simulink model "QuadSE3TrajLinFilt"  (R2017b)
settings: Solver=ode4  StartTime=0.0  StopTime=20  FixedStep=sim_step  RelTol=1e-3  EnableMultiTasking=on
values from neighbouring files (symbols this model uses):
  g = 9.81    [initNH.m]
  initlinvel = zeros(3,1)    [initNH.m]
  initpos = zeros(3,1)    [initNH.m]
  initRotMat = eye(3)    [initNH.m]
  initrotvel = zeros(3,1)    [initNH.m]
  J = diag([0.557, 0.557, 1.05]*10e-2)    [initNH.m]
  kd = 1.4*sqrt(4*kp)    [initNH.m]
  kd_z = kd    [initNH.m]
  KDP = 20    [initNH.m]
  KDR = 20    [initNH.m]
  KDY = 10    [initNH.m]
  ki = 1    [initNH.m]
  kp = 15    [initNH.m]
  KPP = 100    [initNH.m]
  KPR = 100    [initNH.m]
  m = 0.5    [initNH.m]
  max_pos_err_norm = 10    [initNH.m]
  max_tilt = 45/180*pi    (= 0.785398163397)    [initNH.m]
settings Model: Creator=Burak  LastModifiedBy=buyue
settings DataIOCC: LimitDataPoints=on  SaveFormat=Array
settings OptimizationCC: LifeSpan=inf
settings DebuggingCC: UnderspecifiedInitializationDetection=Classic  MergeDetectMultiDrivingBlocksExec=none  SolverPrmCheckMsg=warning  StateNameClashWarn=warning  SFUnexpectedBacktrackingDiag=warning  SFNoUnconditionalDefaultTransitionDiag=warning  SFExecutionAtInitializationDiag=none
settings HardwareCC: ProdBitPerPointer=32  ProdBitPerSizeT=32  ProdBitPerPtrDiffT=32  ProdLargestAtomicFloat=None  ProdIntDivRoundTo=Undefined  ProdEndianess=Unspecified  ProdWordSize=32  ProdHWDeviceType=32-bit Generic
settings ModelReferenceCC: PropagateSignalLabelsOutOfModel=off
settings CodeAppCC: StateflowObjectComments=on
settings GRTTargetCC: TargetLangStandard=C89/C90 (ANSI)  GeneratePreprocessorConditionals=Disable all
settings ConfigComp: CovMetricSettings=dw  CovHtmlReporting=on  CovSaveCumulativeToWorkspaceVar=on  CovSaveSingleToWorkspaceVar=on  CovExternalEMLEnable=off

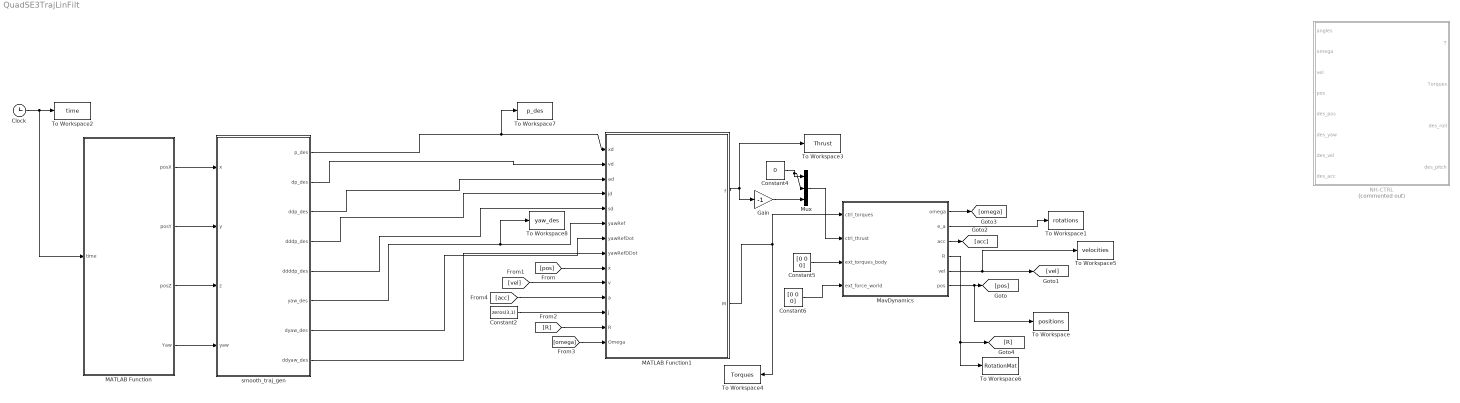
== system QuadSE3TrajLinFilt ==
  Clock : Clock
  Constant2 : Constant  Value=zeros(3,1)
  Constant4 : Constant  Value=0
  Constant5 : Constant  Value=[0 0 0]
  Constant6 : Constant  Value=[0 0 0]
  Gain : Gain  Gain=-1
  MATLAB Function : MATLAB Function  TreatAsAtomicUnit=on
  MATLAB Function1 : MATLAB Function  TreatAsAtomicUnit=on
  MavDynamics : Subsystem
  Mux : Mux  Inputs=3
  NH-CTRL : Subsystem  Commented=on
  To Workspace : ToWorkspace  VariableName=positions  SampleTime=-1
  To Workspace1 : ToWorkspace  VariableName=rotations  SampleTime=-1
  To Workspace2 : ToWorkspace  VariableName=time  SampleTime=-1
  To Workspace3 : ToWorkspace  VariableName=Thrust  SampleTime=-1
  To Workspace4 : ToWorkspace  VariableName=Torques  SampleTime=-1
  To Workspace5 : ToWorkspace  VariableName=velocities  SampleTime=-1
  To Workspace6 : ToWorkspace  VariableName=RotationMat  SampleTime=-1
  To Workspace7 : ToWorkspace  VariableName=p_des  SampleTime=-1
  To Workspace8 : ToWorkspace  VariableName=yaw_des  SampleTime=-1
  smooth_traj_gen : Subsystem
  wires:
  [R] -> MATLAB Function1/13(R)
  [omega] -> MATLAB Function1/14(Omega)
  [pos] -> MATLAB Function1/9(x)
  [vel] -> MATLAB Function1/10(v)
  MATLAB Function1/2(M) -> To Workspace4/1, MavDynamics/1(ctrl_torques)
  MATLAB Function1/1(f) -> Gain/1, To Workspace3/1
  MavDynamics/2(e_a) -> To Workspace1/1
  MavDynamics/5(vel) -> To Workspace5/1, [vel]
  MavDynamics/6(pos) -> To Workspace/1, [pos]
  MavDynamics/1(omega) -> [omega]
  Constant5/1 -> MavDynamics/3(ext_torques_body)
  Constant6/1 -> MavDynamics/4(ext_force_world)
  MavDynamics/4(R) -> [R], To Workspace6/1
  smooth_traj_gen/4(dddp_des) -> MATLAB Function1/4(jd)
  smooth_traj_gen/5(ddddp_des) -> MATLAB Function1/5(sd)
  smooth_traj_gen/7(dyaw_des) -> MATLAB Function1/7(yawRefDot)
  smooth_traj_gen/8(ddyaw_des) -> MATLAB Function1/8(yawRefDDot)
  Clock/1 -> MATLAB Function/1(time), To Workspace2/1
  MATLAB Function/1(posX) -> smooth_traj_gen/1(x)
  MATLAB Function/2(posY) -> smooth_traj_gen/2(y)
  MATLAB Function/3(posZ) -> smooth_traj_gen/3(z)
  MATLAB Function/4(Yaw) -> smooth_traj_gen/4(yaw)
  smooth_traj_gen/3(ddp_des) -> MATLAB Function1/3(ad)
  smooth_traj_gen/2(dp_des) -> MATLAB Function1/2(vd)
  smooth_traj_gen/1(p_des) -> To Workspace7/1, MATLAB Function1/1(xd)
  smooth_traj_gen/6(yaw_des) -> To Workspace8/1, MATLAB Function1/6(yawRef)
  MavDynamics/3(acc) -> [acc]
  [acc] -> MATLAB Function1/11(a)
  Mux/1 -> MavDynamics/2(ctrl_thrust)
  Constant4/1 -> Mux/2, Mux/1
  Gain/1 -> Mux/3
  Constant2/1 -> MATLAB Function1/12(j)

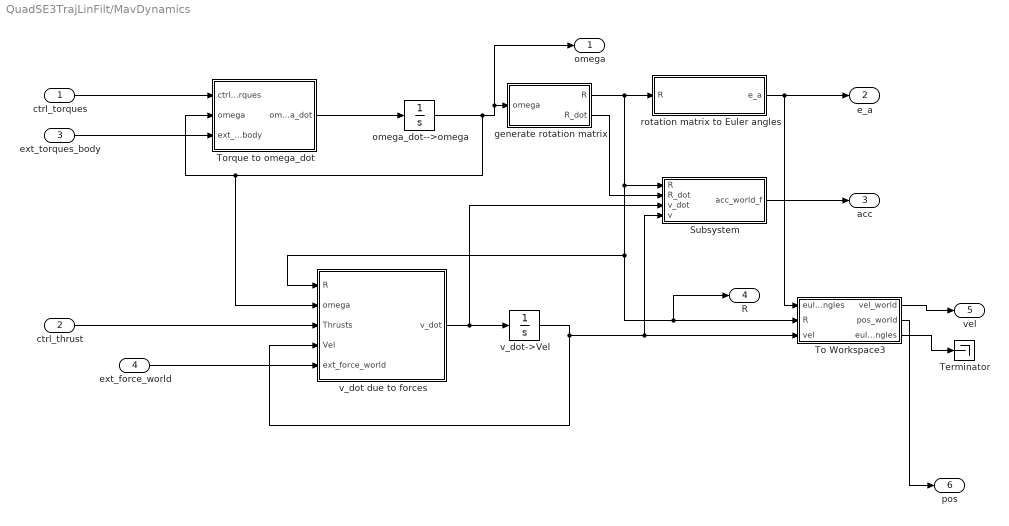
== system QuadSE3TrajLinFilt/MavDynamics ==
  ctrl_torques : Inport
  ctrl_thrust : Inport  Port=2
  ext_torques_body : Inport  Port=3
  ext_force_world : Inport  Port=4
  Subsystem : Subsystem
  Terminator : Terminator
  To Workspace3 : Subsystem
  Torque to omega_dot : Subsystem
  generate rotation matrix : Subsystem
  omega_dot-->omega : Integrator  InitialCondition=initrotvel
  rotation matrix to Euler angles : MATLAB Function  TreatAsAtomicUnit=on
  v_dot due to forces : Subsystem
  v_dot->Vel : Integrator  InitialCondition=initlinvel
  omega : Outport
  e_a : Outport  Port=2
  acc : Outport  Port=3
  R : Outport  Port=4
  vel : Outport  Port=5
  pos : Outport  Port=6
  wires:
  To Workspace3/3("euler_angles ") -> Terminator/1
  v_dot due to forces/1(v_dot) -> Subsystem/3(v_dot), v_dot->Vel/1
  omega_dot-->omega/1 -> v_dot due to forces/2(omega), Torque to omega_dot/2(omega), omega/1, generate rotation matrix/1(omega)
  ext_force_world/1 -> v_dot due to forces/5(ext_force_world)
  To Workspace3/2(pos_world) -> pos/1
  Subsystem/1(acc_world_f) -> acc/1
  To Workspace3/1(vel_world) -> vel/1
  ctrl_thrust/1 -> v_dot due to forces/3(Thrusts)
  rotation matrix to Euler angles/1(e_a) -> e_a/1, To Workspace3/1(euler_angles)
  ext_torques_body/1 -> Torque to omega_dot/3(ext_torques_body)
  Torque to omega_dot/1(omega_dot) -> omega_dot-->omega/1
  generate rotation matrix/1(R) -> rotation matrix to Euler angles/1(R), R/1, To Workspace3/2(R), v_dot due to forces/1(R), Subsystem/1(R)
  v_dot->Vel/1 -> To Workspace3/3(vel), Subsystem/4(v), v_dot due to forces/4(Vel)
  generate rotation matrix/2(R_dot) -> Subsystem/2(R_dot)
  ctrl_torques/1 -> Torque to omega_dot/1(ctrl_orques)

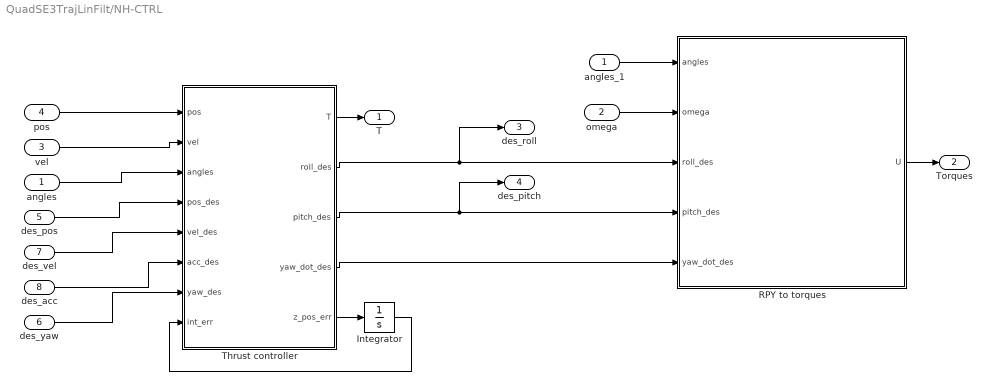
== system QuadSE3TrajLinFilt/NH-CTRL ==
  angles : Inport
  omega : Inport  Port=2
  vel : Inport  Port=3
  pos : Inport  Port=4
  des_pos : Inport  Port=5
  des_yaw : Inport  Port=6
  des_vel : Inport  Port=7
  des_acc : Inport  Port=8
  Integrator : Integrator
  RPY to torques : MATLAB Function  TreatAsAtomicUnit=on
  Thrust controller : MATLAB Function  TreatAsAtomicUnit=on
  angles_1 : InportShadow
  T : Outport
  Torques : Outport  Port=2
  des_roll : Outport  Port=3
  des_pitch : Outport  Port=4
  wires:
  Integrator/1 -> Thrust controller/8(int_err)
  omega/1 -> RPY to torques/2(omega)
  vel/1 -> Thrust controller/2(vel)
  Thrust controller/3(pitch_des) -> des_pitch/1, RPY to torques/4(pitch_des)
  Thrust controller/4(yaw_dot_des) -> RPY to torques/5(yaw_dot_des)
  angles_1/1 -> RPY to torques/1(angles)
  des_acc/1 -> Thrust controller/6(acc_des)
  des_pos/1 -> Thrust controller/4(pos_des)
  des_yaw/1 -> Thrust controller/7(yaw_des)
  pos/1 -> Thrust controller/1(pos)
  Thrust controller/2(roll_des) -> des_roll/1, RPY to torques/3(roll_des)
  angles/1 -> Thrust controller/3(angles)
  Thrust controller/5(z_pos_err) -> Integrator/1
  des_vel/1 -> Thrust controller/5(vel_des)
  RPY to torques/1(U) -> Torques/1
  Thrust controller/1(T) -> T/1

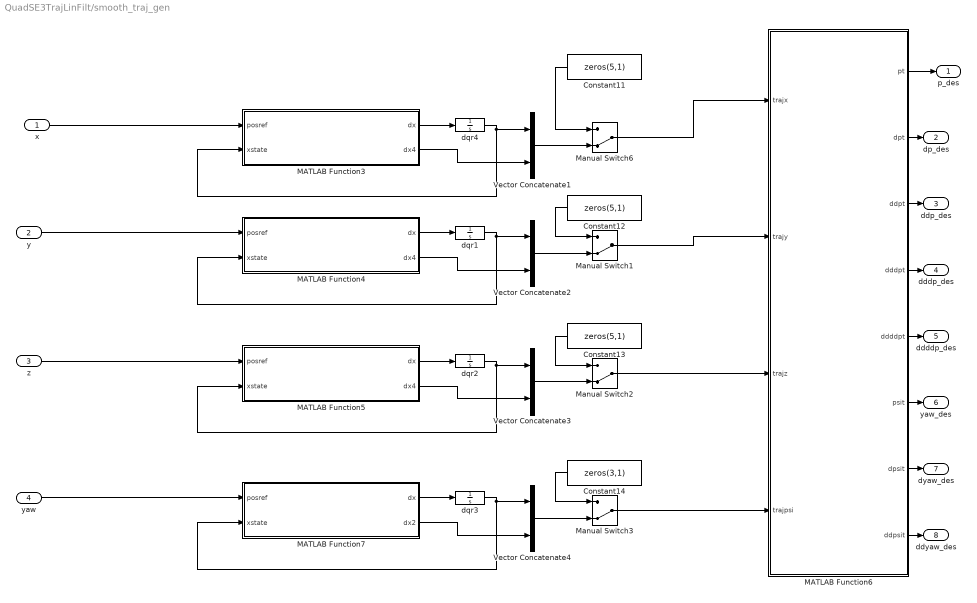
== system QuadSE3TrajLinFilt/smooth_traj_gen ==
  x : Inport
  y : Inport  Port=2
  z : Inport  Port=3
  yaw : Inport  Port=4
  Constant11 : Constant  Value=zeros(5,1)
  Constant12 : Constant  Value=zeros(5,1)
  Constant13 : Constant  Value=zeros(5,1)
  Constant14 : Constant  Value=zeros(3,1)
  MATLAB Function3 : MATLAB Function  TreatAsAtomicUnit=on
  MATLAB Function4 : MATLAB Function  TreatAsAtomicUnit=on
  MATLAB Function5 : MATLAB Function  TreatAsAtomicUnit=on
  MATLAB Function6 : MATLAB Function  TreatAsAtomicUnit=on
  MATLAB Function7 : MATLAB Function  TreatAsAtomicUnit=on
  Manual Switch{1..3,6} (4 alike) : ManualSwitch  CurrentSetting=0
  Vector Concatenate{1..4} (4 alike) : Concatenate
  dqr1 : Integrator  InitialCondition=[0,0,0,0];
  dqr2 : Integrator  InitialCondition=[0,0,0,0];
  dqr3 : Integrator  InitialCondition=[0,0];
  dqr4 : Integrator  InitialCondition=[0,0,0,0];
  p_des : Outport
  dp_des : Outport  Port=2
  ddp_des : Outport  Port=3
  dddp_des : Outport  Port=4
  ddddp_des : Outport  Port=5
  yaw_des : Outport  Port=6
  dyaw_des : Outport  Port=7
  ddyaw_des : Outport  Port=8
  wires:
  MATLAB Function6/1(pt) -> p_des/1
  MATLAB Function7/2(dx2) -> Vector Concatenate4/2
  x/1 -> MATLAB Function3/1(posref)
  dqr2/1 -> Vector Concatenate3/1, MATLAB Function5/2(xstate)
  MATLAB Function3/1(dx) -> dqr4/1
  MATLAB Function7/1(dx) -> dqr3/1
  yaw/1 -> MATLAB Function7/1(posref)
  MATLAB Function5/2(dx4) -> Vector Concatenate3/2
  Constant14/1 -> Manual Switch3/1
  Manual Switch3/1 -> MATLAB Function6/4(trajpsi)
  MATLAB Function4/1(dx) -> dqr1/1
  MATLAB Function3/2(dx4) -> Vector Concatenate1/2
  MATLAB Function5/1(dx) -> dqr2/1
  Constant13/1 -> Manual Switch2/1
  MATLAB Function4/2(dx4) -> Vector Concatenate2/2
  Vector Concatenate2/1 -> Manual Switch1/2
  Vector Concatenate1/1 -> Manual Switch6/2
  Constant11/1 -> Manual Switch6/1
  Vector Concatenate3/1 -> Manual Switch2/2
  Manual Switch6/1 -> MATLAB Function6/1(trajx)
  Constant12/1 -> Manual Switch1/1
  Manual Switch1/1 -> MATLAB Function6/2(trajy)
  y/1 -> MATLAB Function4/1(posref)
  z/1 -> MATLAB Function5/1(posref)
  dqr3/1 -> Vector Concatenate4/1, MATLAB Function7/2(xstate)
  dqr4/1 -> Vector Concatenate1/1, MATLAB Function3/2(xstate)
  dqr1/1 -> Vector Concatenate2/1, MATLAB Function4/2(xstate)
  Vector Concatenate4/1 -> Manual Switch3/2
  Manual Switch2/1 -> MATLAB Function6/3(trajz)
  MATLAB Function6/4(dddpt) -> dddp_des/1
  MATLAB Function6/2(dpt) -> dp_des/1
  MATLAB Function6/5(ddddpt) -> ddddp_des/1
  MATLAB Function6/6(psit) -> yaw_des/1
  MATLAB Function6/8(ddpsit) -> ddyaw_des/1
  MATLAB Function6/7(dpsit) -> dyaw_des/1
  MATLAB Function6/3(ddpt) -> ddp_des/1

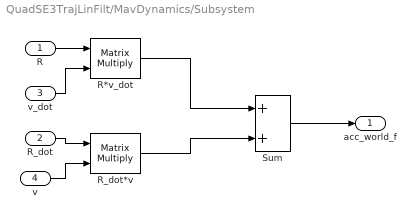
== system QuadSE3TrajLinFilt/MavDynamics/Subsystem ==
  R : Inport
  R_dot : Inport  Port=2
  v_dot : Inport  Port=3
  v : Inport  Port=4
  R*v_dot : Product  Multiplication=Matrix(*)  RndMeth=Zero
  R_dot*v : Product  Multiplication=Matrix(*)  RndMeth=Zero
  Sum : Sum
  acc_world_f : Outport
  wires:
  Sum/1 -> acc_world_f/1
  R/1 -> R*v_dot/1
  v_dot/1 -> R*v_dot/2
  R_dot/1 -> R_dot*v/1
  v/1 -> R_dot*v/2
  R*v_dot/1 -> Sum/1
  R_dot*v/1 -> Sum/2

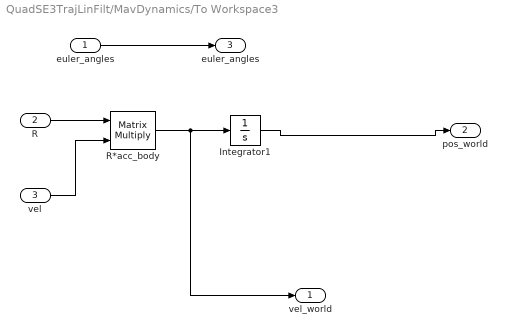
== system QuadSE3TrajLinFilt/MavDynamics/To Workspace3 ==
  euler_angles : Inport
  R : Inport  Port=2
  vel : Inport  Port=3
  Integrator1 : Integrator  InitialCondition=initpos
  R*acc_body : Product  Multiplication=Matrix(*)  RndMeth=Zero
  vel_world : Outport
  pos_world : Outport  Port=2
  "euler_angles " : Outport  Port=3
  wires:
  R/1 -> R*acc_body/1
  vel/1 -> R*acc_body/2
  euler_angles/1 -> "euler_angles "/1
  R*acc_body/1 -> vel_world/1, Integrator1/1
  Integrator1/1 -> pos_world/1

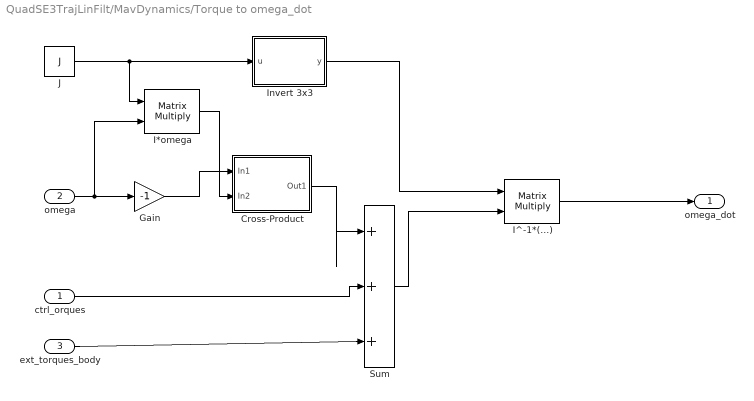
== system QuadSE3TrajLinFilt/MavDynamics/Torque to omega_dot ==
  ctrl_orques : Inport
  omega : Inport  Port=2
  ext_torques_body : Inport  Port=3
  Cross-Product : Subsystem
  Gain : Gain  Gain=-1
  I*omega : Product  Multiplication=Matrix(*)  RndMeth=Zero
  I^-1*(...) : Product  Multiplication=Matrix(*)  RndMeth=Zero
  Invert 3x3 : MATLAB Function  TreatAsAtomicUnit=on
  J : Constant  Value=J
  Sum : Sum  Inputs=|+++
  omega_dot : Outport
  wires:
  omega/1 -> I*omega/2, Gain/1
  J/1 -> I*omega/1, Invert 3x3/1(u)
  I*omega/1 -> Cross-Product/2(In2)
  Invert 3x3/1(y) -> I^-1*(...)/1
  I^-1*(...)/1 -> omega_dot/1
  ctrl_orques/1 -> Sum/2
  Sum/1 -> I^-1*(...)/2
  Gain/1 -> Cross-Product/1(In1)
  Cross-Product/1(Out1) -> Sum/1
  ext_torques_body/1 -> Sum/3

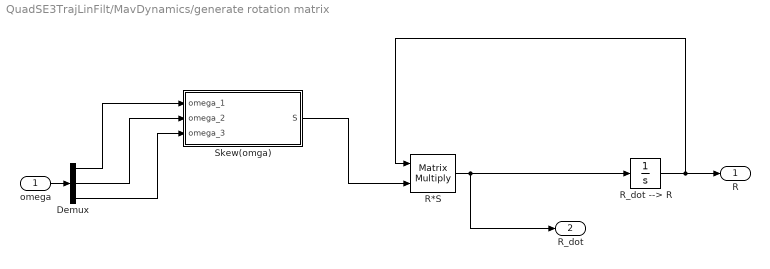
== system QuadSE3TrajLinFilt/MavDynamics/generate rotation matrix ==
  omega : Inport
  Demux : Demux  Outputs=3
  R*S : Product  Multiplication=Matrix(*)  RndMeth=Zero
  R_dot --> R : Integrator  InitialCondition=initRotMat
  Skew(omga) : MATLAB Function  TreatAsAtomicUnit=on
  R : Outport
  R_dot : Outport  Port=2
  wires:
  R*S/1 -> R_dot --> R/1, R_dot/1
  R_dot --> R/1 -> R/1, R*S/1
  omega/1 -> Demux/1
  Demux/1 -> Skew(omga)/1(omega_1)
  Demux/2 -> Skew(omga)/2(omega_2)
  Demux/3 -> Skew(omga)/3(omega_3)
  Skew(omga)/1(S) -> R*S/2

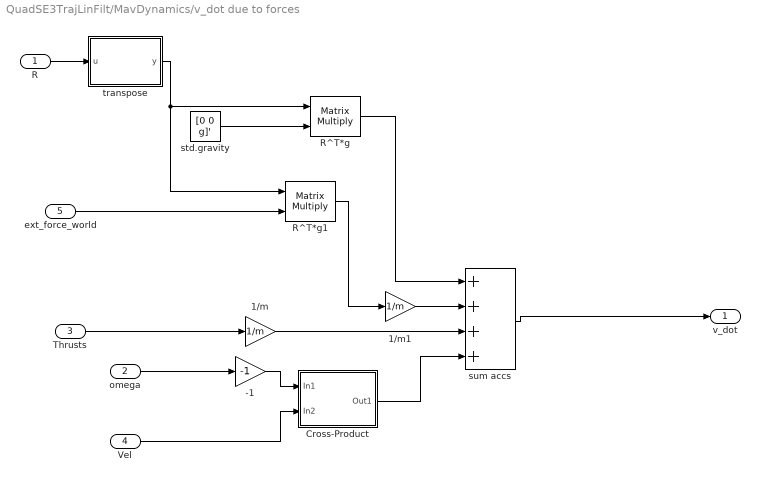
== system QuadSE3TrajLinFilt/MavDynamics/v_dot due to forces ==
  R : Inport
  omega : Inport  Port=2
  Thrusts : Inport  Port=3
  Vel : Inport  Port=4
  ext_force_world : Inport  Port=5
  -1 : Gain  Gain=-1
  1/m : Gain  Gain=1/m
  1/m1 : Gain  Gain=1/m
  Cross-Product : Subsystem
  R^T*g : Product  Multiplication=Matrix(*)  RndMeth=Zero
  R^T*g1 : Product  Multiplication=Matrix(*)  RndMeth=Zero
  std.gravity : Constant  Value=[0 0 g]'
  sum accs : Sum  Inputs=++++
  transpose : MATLAB Function  TreatAsAtomicUnit=on
  v_dot : Outport
  wires:
  omega/1 -> -1/1
  Vel/1 -> Cross-Product/2(In2)
  R/1 -> transpose/1(u)
  transpose/1(y) -> R^T*g1/1, R^T*g/1
  std.gravity/1 -> R^T*g/2
  R^T*g/1 -> sum accs/1
  sum accs/1 -> v_dot/1
  Thrusts/1 -> 1/m/1
  -1/1 -> Cross-Product/1(In1)
  Cross-Product/1(Out1) -> sum accs/4
  1/m/1 -> sum accs/3
  ext_force_world/1 -> R^T*g1/2
  R^T*g1/1 -> 1/m1/1
  1/m1/1 -> sum accs/2

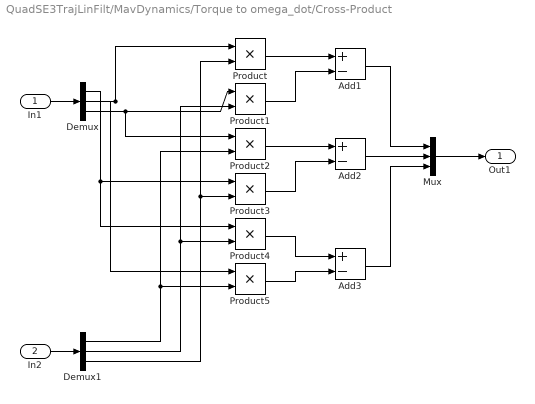
== system QuadSE3TrajLinFilt/MavDynamics/Torque to omega_dot/Cross-Product ==
  In1 : Inport
  In2 : Inport  Port=2
  Add1 : Sum  Inputs=+-
  Add2 : Sum  Inputs=+-
  Add3 : Sum  Inputs=+-
  Demux : Demux  Outputs=3
  Demux1 : Demux  Outputs=3
  Mux : Mux  Inputs=3
  Product{,1..5} (6 alike) : Product  RndMeth=Zero
  Out1 : Outport
  wires:
  In1/1 -> Demux/1
  In2/1 -> Demux1/1
  Mux/1 -> Out1/1
  Add1/1 -> Mux/1
  Add2/1 -> Mux/2
  Add3/1 -> Mux/3
  Demux/2 -> Product/1, Product5/1
  Demux1/3 -> Product/2, Product3/2
  Demux/3 -> Product1/1, Product2/1
  Demux1/2 -> Product1/2, Product4/2
  Demux/1 -> Product3/1, Product4/1
  Demux1/1 -> Product2/2, Product5/2
  Product/1 -> Add1/1
  Product1/1 -> Add1/2
  Product2/1 -> Add2/1
  Product3/1 -> Add2/2
  Product4/1 -> Add3/1
  Product5/1 -> Add3/2

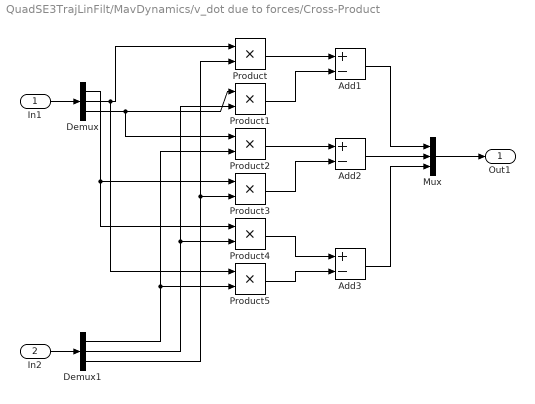
== system QuadSE3TrajLinFilt/MavDynamics/v_dot due to forces/Cross-Product ==
  In1 : Inport
  In2 : Inport  Port=2
  Add1 : Sum  Inputs=+-
  Add2 : Sum  Inputs=+-
  Add3 : Sum  Inputs=+-
  Demux : Demux  Outputs=3
  Demux1 : Demux  Outputs=3
  Mux : Mux  Inputs=3
  Product{,1..5} (6 alike) : Product  RndMeth=Zero
  Out1 : Outport
  wires:
  In1/1 -> Demux/1
  In2/1 -> Demux1/1
  Mux/1 -> Out1/1
  Add1/1 -> Mux/1
  Add2/1 -> Mux/2
  Add3/1 -> Mux/3
  Demux/2 -> Product/1, Product5/1
  Demux1/3 -> Product/2, Product3/2
  Demux/3 -> Product1/1, Product2/1
  Demux1/2 -> Product1/2, Product4/2
  Demux/1 -> Product3/1, Product4/1
  Demux1/1 -> Product2/2, Product5/2
  Product/1 -> Add1/1
  Product1/1 -> Add1/2
  Product2/1 -> Add2/1
  Product3/1 -> Add2/2
  Product4/1 -> Add3/1
  Product5/1 -> Add3/2

== matlab function QuadSE3TrajLinFilt/MATLAB Function1 ==
  data: xd input; f output; vd input; ad input; jd input; sd input; yawRef input; yawRefDot input; yawRefDDot input; x input; v input; a input; j input; R input; Omega input; J parameter; g parameter; M output; m parameter
function [f, M] = SE3Ctrl(xd,vd,ad,jd,sd,yawRef,yawRefDot,yawRefDDot,x,v,a,j,R,Omega,J, g, m)
% control gains
kx = 4*m;
kv = 5.6*m;
kR = 8.81;
kOmega = 2.54;
% calculate translational errors
error_x = x - xd;
error_v = v - vd;
error_a = a - ad;
error_j = j - jd;
% desired heading as function of yaw and its derivatives     
b1_d      = [cos(yawRef) sin(yawRef) 0]'; %e1
b1_d_dot  = [-sin(yawRef)*yawRefDot cos(yawRef)*yawRefDot 0]';
b1_d_ddot = [-sin(yawRef)*yawRefDDot - cos(yawRef)*yawRefDot^2  cos(yawRef)*yawRefDDot - sin(yawRef)*yawRefDot^2 0]';    
% inertial frame 3-axis
e3 = [0;0;1];
% control thrust and its magnitude
A = -kx*error_x - kv*error_v - m*g*e3 + m*ad;
f = vec_dot(-A, R*e3);
% Now we are going to construct the desired/control rotation matrix
% direction of the thrust vector (desired/control)
% aka body z direction
b3_c = -A/norm(A);
% vector orthogonal to thrust direction and desired heading.
% this is directing to y axis
C = vec_cross(b3_c, b1_d);
% orthonormal desired body y direction
b2_c = C/norm(C);
% orthonormal desired body x direction
b1_c = vec_cross(b2_c,b3_c);
% construct the rotation matrix to be tracked
R_c = [b1_c b2_c b3_c];
% time derivatives of body axes for excessive attitude tracking
% performances
A_dot   = -kx*error_v - kv*error_a + m*jd;
% time derivative of body z
b3_c_dot = -A_dot/norm(A) + (vec_dot(A,A_dot)/norm(A)^3)*A;
C_dot   = vec_cross(b3_c_dot, b1_d) + vec_cross(b3_c, b1_d_dot);
% time derivative of body y
b2_c_dot = C/norm(C) - (vec_dot(C,C_dot)/norm(C)^3)*C;
% time derivative of body x
b1_c_dot = vec_cross(b2_c_dot, b3_c) + vec_cross(b2_c, b3_c_dot);
% second time derivatives of body axes
A_ddot   = -kx*error_a - kv*error_j + m*sd;
% second time derivative of body z
b3_c_ddot = -A_ddot/norm(A) + (2/norm(A)^3)*vec_dot(A,A_dot)*A_dot ...
         + ((norm(A_dot)^2 + vec_dot(A,A_ddot))/norm(A)^3)*A       ...
         - (3/norm(A)^5)*(vec_dot(A,A_dot)^2)*A;
C_ddot   = vec_cross(b3_c_ddot, b1_d) + vec_cross(b3_c, b1_d_ddot)          ...
         + 2*vec_cross(b3_c_dot, b1_d_dot);
% time derivative of body y
b2_c_ddot = C_ddot/norm(C) - (2/norm(C)^3)*vec_dot(C,C_dot)*C_dot  ...
         - ((norm(C_ddot)^2 + vec_dot(C,C_ddot))/norm(C)^3)*C       ...
         + (3/norm(C)^5)*(vec_dot(C,C_dot)^2)*C;
% time derivative of body x
b1_c_ddot = vec_cross(b2_c_ddot, b3_c) + vec_cross(b2_c, b3_c_ddot)          ...
         + 2*vec_cross(b2_c_dot, b3_c_dot);
% High order rotation terms
R_c_dot      = [b1_c_dot b2_c_dot b3_c_dot];
R_c_ddot     = [b1_c_ddot b2_c_ddot b3_c_ddot];
Omega_c      = vee(R_c'*R_c_dot);
Omega_c_dot  = vee(R_c'*R_c_ddot - hat(Omega_c)*hat(Omega_c));
% proper error definition in SO3 and in its tangent
error_R     = (1/2)*vee(R_c.'*R - R.'*R_c);
error_Omega = Omega - R.'*R_c*Omega_c;
% % disturb J
% J = J + J*1.2;
% control torques
M = -kR*error_R - kOmega*error_Omega + vec_cross(Omega, J*Omega) ...
  - J*(hat(Omega)*R.'*R_c*Omega_c - R.'*R_c*Omega_c_dot);
    
end

function c = vec_cross(a, b)
    c = [a(2)*b(3) - a(3)*b(2) ;
         -a(1)*b(3) + a(3)*b(1) ;
         a(1)*b(2) - a(2)*b(1)] ;
end

function t = vee(A)
t = [A(3,2) ;
     A(1,3) ;
     A(2,1)] ;
end

function A = hat(t)
    A = [0 -t(3) t(2) ; t(3) 0 -t(1) ; -t(2) t(1) 0] ;
end

function c = vec_dot(a, b)
    c = a'*b ;
end

== matlab function QuadSE3TrajLinFilt/MATLAB Function ==
  data: time input; posX output; posY output; posZ output; Yaw output
function [posX, posY, posZ, Yaw] = genPoints(time)
posX = 1;
posY = 1;
posZ = 1;
Yaw  = 1;
%% Spiral
% posX = 4*sin(time);
% posY = 4*cos(time);
% posZ = -0.75*time;
% Yaw  = -time;
%% Ramp 3D
% posX = 0.5*time;
% posY = 0.5*time;
% posZ = -time;
% Yaw = 0;
%% Generic
% posX = 0;
% posY = 0;
% posZ = 0;
% Yaw  = 0;
% if time >0.1 && time<5.0
%     posZ = -5;
%     Yaw = pi/2;
% elseif time >=5.0 && time<10.0
%     posZ = -5;
%     posY = 5;
%     Yaw = pi/2;
% end

== matlab function QuadSE3TrajLinFilt/NH-CTRL/RPY to torques ==
  data: angles input; U output; omega input; roll_des input; pitch_des input; yaw_dot_des input; J parameter; KDR parameter; KPR parameter; KDP parameter; KPP parameter; KDY parameter
function U  = fcn(angles, omega, roll_des, pitch_des, yaw_dot_des, J, KDR, KPR, KDP, KPP, KDY)
% This block supports the Embedded MATLAB subset.
% See the help menu for details. 

% p = angles(2);
% r = angles(1);
% y=angles(3);
% 
% T = [1      tan(p)*sin(r) tan(p)*cos(r);
%     0       cos(r)  -sin(r);
%     0       sin(r)/cos(p)   cos(r)/cos(p)];
% 
% dot_ang = T*omega;
% dot_r=dot_ang(1);
% dot_p = dot_ang(2);
% 
% T_dot = [0  tan(p)*cos(r)*dot_r+(sin(r)+tan(p)^2*sin(r))*dot_p -tan(p)*sin(r)*dot_r+(cos(r)+tan(p)^2*cos(r))*dot_p;
%          0  -sin(r)*dot_r   -cos(r)*dot_r;
%          0  cos(r)/cos(p)*dot_r+sin(r)*sin(p)/cos(p)^2*dot_p    -sin(r)/cos(p)*dot_r+cos(r)*sin(p)/cos(p)^2*dot_p];
% 
% 
% k_d = 11;
% k_p = 30;
% ang_vel_des = [0 0 yaw_dot_des]';
% 
% 
% if(yaw_des - angles(3) > pi)
%     angles(3) = angles(3)+2*pi;
% elseif (yaw_des - angles(3) < -pi)
%     angles(3) = angles(3)-2*pi;
% end
% 
% ang_des = [roll_des pitch_des yaw_des]';
% U = I*inv(T)*(k_d*(ang_vel_des-dot_ang)+k_p*(ang_des - angles)-T_dot*omega)+cross(omega, I*omega);
% r_c = U(1);
% p_c = U(2);
% y_c = U(3);

U=[0;0;0];

r = angles(1);
p = angles(2);
y=angles(3);


T = [1      tan(p)*sin(r) tan(p)*cos(r);
    0       cos(r)  -sin(r);
    0       sin(r)/cos(p)   cos(r)/cos(p)];

dot_ang = T*omega;

dot_r= dot_ang(1);
dot_p = dot_ang(2);
dot_y = dot_ang(3);



% KDR = 20; 
% KPR = 100;
% 
% KDP = 20; 
% KPP = 100;
% 
% 
% KDY = 10;
% % KPY = 5;

Sw = [0 -omega(3) omega(2);                         % hat operation: R3->so3 (inverse of vee)
      omega(3) 0 -omega(1);
     -omega(2) omega(1) 0];

U=Sw*J*omega + J*inv(T)*([ KDR * (0 - dot_r) + KPR * (roll_des - r); KDP * (0 - dot_p) + KPP * (pitch_des - p) ; KDY * (yaw_dot_des - dot_y) ]);
% U=J*inv(T)*([ KDR * (0 - dot_r) + KPR * (roll_des - r); KDP * (0 - dot_p) + KPP * (pitch_des - p) ; KDY * (yaw_dot_des - dot_y) ]);


% U(1) = KDR * (0 - dot_r) + KPR * (roll_des - r);
% U(2) = KDP * (0 - dot_p) + KPP * (pitch_des - p);
% U(3) = KDY * (yaw_dot_des - dot_y);  %+ KPY * (yaw_des - y);
% 
% U=J*U;

== matlab function QuadSE3TrajLinFilt/NH-CTRL/Thrust controller ==
  data: pos input; vel input; angles input; pos_des input; g parameter; m parameter; T output; roll_des output; pitch_des output; vel_des input; acc_des input; yaw_des input; yaw_dot_des output; kd parameter; kp parameter; ki parameter; max_tilt parameter; kd_z parameter; max_pos_err_norm parameter; int_err input; z_pos_err output
function [T, roll_des, pitch_des, yaw_dot_des,z_pos_err] = fcn(pos, vel, angles, pos_des, g, m, vel_des, acc_des,yaw_des, kd, kp, ki, max_tilt, kd_z, max_pos_err_norm,int_err)

r = angles(1);
p = angles(2);
y = angles(3);

pos_err = pos_des-pos;
T=zeros(3,1);

%hard saturation
% if norm(pos_err)>max_pos_err_norm
%     pos_err=pos_err/norm(pos_err)*max_pos_err_norm;
% end

%soft saturation
sat_norm = (2*max_pos_err_norm/pi) * atan( pi* norm(pos_err) / (2*max_pos_err_norm) );
if norm(pos_err) > 0.0001
    pos_err = pos_err/norm(pos_err) * sat_norm;
end

T=[0;0;m/(cos(r)*cos(p))*(-g+ acc_des(3) + kd_z*(vel_des(3) -vel(3)) + kp*(pos_err(3)) +ki*int_err )];


ddpx=kd*(vel_des(1) -vel(1)) + kp*(pos_err(1));
ddpy=kd*(vel_des(2) -vel(2)) + kp*(pos_err(2));

max_roll=sin(max_tilt);
max_pitch=sin(max_tilt);


ctrl_roll=m/T(3)*( -sin(y)*ddpx+cos(y)*ddpy);
ctrl_pitch= m/(T(3)*cos(r))*( cos(y)*ddpx+sin(y)*ddpy);


%hard saturation
% if abs(ctrl_roll)>max_roll
%     ctrl_roll=sign(ctrl_roll)*max_roll;
%     angle_sat=1;
% end
% 
% if abs(ctrl_pitch)>max_pitch
%     ctrl_pitch=sign(ctrl_pitch)*max_pitch;
%     angle_sat=1;
% end

%soft saturation
ctrl_roll = (2*max_roll/pi) * atan( pi* ctrl_roll / (2*max_roll) );

ctrl_pitch = (2*max_pitch/pi) * atan( pi* ctrl_pitch / (2*max_pitch) );

roll_des = -asin(ctrl_roll);

pitch_des = asin(ctrl_pitch);


% saturation
% if abs(roll_des) > max_tilt
%     
%     roll_des = sign(roll_des)*max_tilt;
%     
% end
% if abs(pitch_des) > max_tilt
%     
%     pitch_des = sign(pitch_des)*max_tilt;
%     
% end

z_pos_err = pos_err(3);

yaw_dot_des = kp*atan2(sin(yaw_des-y),cos(yaw_des-y));

== matlab function QuadSE3TrajLinFilt/MavDynamics/Torque to omega_dot/Invert 3x3 ==
  data: u input; y output
function y = fcn(u)


y = NaN(3,3);
y(1,1) = u(3,3)*u(2,2)- u(2,3)*u(3,2);
y(1,2) = u(1,3)*u(3,2)- u(3,3)*u(1,2);
y(1,3) = u(1,2)*u(2,3)- u(2,2)*u(1,3);

y(2,1) = u(2,3)*u(3,1)- u(2,1)*u(3,3);
y(2,2) = u(1,1)*u(3,3)- u(3,1)*u(1,3);
y(2,3) = u(1,3)*u(2,1)- u(1,1)*u(2,3);

y(3,1) = u(2,1)*u(3,2)- u(2,2)*u(3,1);
y(3,2) = u(1,2)*u(3,1)- u(1,1)*u(3,2);
y(3,3) = u(1,1)*u(2,2)- u(1,2)*u(2,1);

y=1/det(u)*y;

== matlab function QuadSE3TrajLinFilt/MavDynamics/generate rotation matrix/Skew(omga) ==
  data: omega_1 input; S output; omega_2 input; omega_3 input
function S = skew(omega_1, omega_2, omega_3)
% This block supports the Embedded MATLAB subset.
% See the help menu for details. 
S = [0 -omega_3 omega_2;
 omega_3 0 -omega_1;
 -omega_2 omega_1 0];

== matlab function QuadSE3TrajLinFilt/MavDynamics/rotation matrix to Euler angles ==
  data: R input; e_a output
function e_a = eulerangles(R)
% This block supports an embeddable subset of the MATLAB language.
% See the help menu for details. 

e_a = zeros(3,1);

Roll = atan2(R(3,2),R(3,3));
Pitch = atan2(-R(3,1),sqrt(R(3,2)^2+R(3,3)^2));
Yaw = atan2(R(2,1),R(1,1));


e_a = [Roll; Pitch; Yaw];

== matlab function QuadSE3TrajLinFilt/MavDynamics/v_dot due to forces/transpose ==
  data: u input; y output
function y = fcn(u)
% This block supports the Embedded MATLAB subset.
% See the help menu for details. 

y = u';

== matlab function QuadSE3TrajLinFilt/smooth_traj_gen/MATLAB Function4 ==
  data: posref input; dx output; xstate input; K_trajy parameter; dx4 output
function [dx,dx4]  = trajectory(posref,xstate,K_trajy)
A=[0 1 0 0; 0 0 1 0; 0 0 0 1; 0 0 0 0];
B=[0 0 0 1]';
dx=(A-B*K_trajy)*(xstate-[posref;0;0;0]);
dx4=dx(4);
end

== matlab function QuadSE3TrajLinFilt/smooth_traj_gen/MATLAB Function3 ==
  data: posref input; dx output; xstate input; K_trajx parameter; dx4 output
function [dx,dx4]  = trajectory(posref,xstate,K_trajx)
A=[0 1 0 0; 0 0 1 0; 0 0 0 1; 0 0 0 0];
B=[0 0 0 1]';
dx=(A-B*K_trajx)*(xstate-[posref;0;0;0]);
dx4=dx(4);
end

== matlab function QuadSE3TrajLinFilt/smooth_traj_gen/MATLAB Function5 ==
  data: posref input; dx output; xstate input; K_trajz parameter; dx4 output
function [dx,dx4]  = trajectory(posref,xstate,K_trajz)
A=[0 1 0 0; 0 0 1 0; 0 0 0 1; 0 0 0 0];
B=[0 0 0 1]';
dx=(A-B*K_trajz)*(xstate-[posref;0;0;0]);
dx4=dx(4);
end

== matlab function QuadSE3TrajLinFilt/smooth_traj_gen/MATLAB Function6 ==
  data: pt output; dpt output; ddpt output; dddpt output; ddddpt output; trajx input; trajy input; trajz input; trajpsi input; psit output; dpsit output; ddpsit output
function [pt, dpt, ddpt, dddpt, ddddpt, psit, dpsit, ddpsit] = trajgen(trajx,trajy,trajz,trajpsi)
pt=zeros(3,1);
dpt=zeros(3,1);
ddpt=zeros(3,1);
dddpt=zeros(3,1);
ddddpt=zeros(3,1);
pt(1) = trajx(1);
pt(2) = trajy(1);
pt(3) = trajz(1);
dpt(1) = trajx(2);
dpt(2) = trajy(2);
dpt(3) = trajz(2);
ddpt(1) = trajx(3);
ddpt(2) = trajy(3);
ddpt(3) = trajz(3);
dddpt(1) = trajx(4);
dddpt(2) = trajy(4);
dddpt(3) = trajz(4);
ddddpt(1) = trajx(5);
ddddpt(2) = trajy(5);
ddddpt(3) = trajz(5);
psit = trajpsi(1);
dpsit = trajpsi(2);
ddpsit = trajpsi(3);

== matlab function QuadSE3TrajLinFilt/smooth_traj_gen/MATLAB Function7 ==
  data: posref input; dx output; xstate input; K_trajpsi parameter; dx2 output
function [dx,dx2]  = trajectory(posref,xstate,K_trajpsi)
A=[0 1 ; 0 0];
B=[0 1]';
dx=(A-B*K_trajpsi)*(xstate-[posref;0]);
dx2=dx(2);
end
